simulink model "WorkingDynamics"  (R2018b)
settings: Solver=FixedStepAuto  StartTime=0.0  StopTime=inf  FixedStep=.001  RelTol=5e-3
model workspace (MAT data in the model file):
  A_mu = 10
  B_reff = 8.386
  Cz = 7766.25
  DCT_Param : struct (value not decoded)
  D_reff = 0.25826
  Downshift_Speeds = [9.5625 12.9375 16.3125 19.6875 23.0625 26.4375 29.8125 33.1875 36.5625 39.9375 43.3125 46.6875 ... (28 elements, 4x7)]
  Pedal_Positions = [0.1 0.4 0.5 0.9]
  SUS : struct (value not decoded)
  Upshift_Speeds = [12.9375 16.3125 19.6875 33 26.4375 29.8125 33.1875 52.5 39.9375 43.3125 46.6875 77.25 ... (28 elements, 4x7)]
  VEH : struct (value not decoded)
  V_o = 16.7
  V_xlow = 1
  WH : struct (value not decoded)
  a = 1.4
  alpha_max = 1.5
  alpha_min = -1.5
  b = 1.8
  c_zo = 209651
  epsilon = 0.1
  h = 0.134
  path : struct (value not decoded)
  pio = 220000
  q_Fcx = 0
  q_Fz2 = 15.4
  q_Fzy = 0
  q_reo = 0.9974
  q_sx1 = -0.007764
  q_sx10 = 0.2824
  q_sx11 = 5.349
  q_sx12 = 0
  q_sx13 = 0
  q_sx14 = 0
  q_sx2 = 1.1915
  q_sx3 = 0.013948
  q_sx4 = 4.912
  q_sx5 = 1.02
  q_sx6 = 22.83
  q_sx7 = 0.7104
  q_sx8 = -0.023393
  q_sx9 = 0.6581
  q_sy1 = 0.00702
  q_sy2 = 0
  q_sy3 = 0.001515
  q_sy4 = 8.514e-05
  q_sy5 = 0
  q_sy6 = 0
  q_sy7 = 0.9008
  q_sy8 = -0.4089
  q_v1 = 0.0007742
  q_v2 = 0.04667
  r_Bx1 = 12.531
  r_Bx2 = 9.532
  r_Bx3 = 0
  r_By1 = 10.615
  r_By2 = 7.705
  r_By3 = 3.433e-06
  r_By4 = 0
  r_Cx1 = 1.019
  r_Cy1 = 1.0585
  r_Ex1 = -0.4487
  r_Ex2 = -0.4726
  r_Ey1 = 0.3132
  r_Ey2 = 7.63e-06
  r_Hx1 = 0.0002374
  r_Hy1 = 0.011646
  r_Hy2 = 7.63e-06
  r_Vy1 = 0.05654
  r_Vy2 = 7.63e-06
  r_Vy3 = 0
  r_Vy4 = 99.9
  r_Vy5 = 2
  r_Vy6 = 15.814
  r_o = 0.3135
  vehWidth = 2
  w = 1
libraries: autolibutils x8, autolibshared x6, robotlib x5, simulink x4, autolibsharedcoupling x3, vehdynlibtirecommon x2, sim3dlib x1, vehdynlibsteering x1, autolibshareddiff x1, autolibsharedtransfixedgear x1, sharedtransform x1, autolibsharedmappedengines x1
(part 6 of 6)

== system WorkingDynamics/Passenger Vehicle/Subsystem7/Longitudinal Wheels 4DOF/Veh2Tire ==
  Axle : Inport
  Brake : Inport  Port=2
  r : Inport  Port=3
  VehVel : Inport  Port=4
  WheelSteer : Inport  Port=5
  Reshape3 : Reshape
  Reshape4 : Reshape
  Unary Minus : UnaryMinus
  Wheel to Body Transform : Subsystem
  T : Outport
  P : Outport  Port=2
  xdotAxle : Outport  Port=3
  ydotAxle : Outport  Port=4
  psidot : Outport  Port=5
  zdotAxle : Outport  Port=6
  wires:
  Brake/1 -> Reshape3/1
  Axle/1 -> Reshape4/1
  Wheel to Body Transform/1(xdotWheel) -> xdotAxle/1  "Vx"
  Wheel to Body Transform/2(ydotWheel) -> ydotAxle/1  "Vy"
  r/1 -> Unary Minus/1
  Reshape4/1 -> T/1
  VehVel/1 -> Wheel to Body Transform/1(VelVeh)
  WheelSteer/1 -> Wheel to Body Transform/2(WheelAngles)
  Wheel to Body Transform/3(zdotWheel) -> zdotAxle/1  "Vz"
  Unary Minus/1 -> psidot/1
  Reshape3/1 -> P/1

== system WorkingDynamics/Passenger Vehicle/Subsystem7/Longitudinal Wheels 4DOF/Velocity and Vertical Load ==
  note: 1) Add Subsystem or Model blocks as valid variant choices.
      | 2) You cannot connect blocks at this level. At simulation, connectivity is automatically
      | determined, based on the active variant and port name matching.
  VehFdbk : Inport
  Bicycle : Subsystem  VariantControl=0
  Dual : Subsystem  VariantControl=1
  VehV : Outport
  Fz : Outport  Port=2  PortDimensions=4

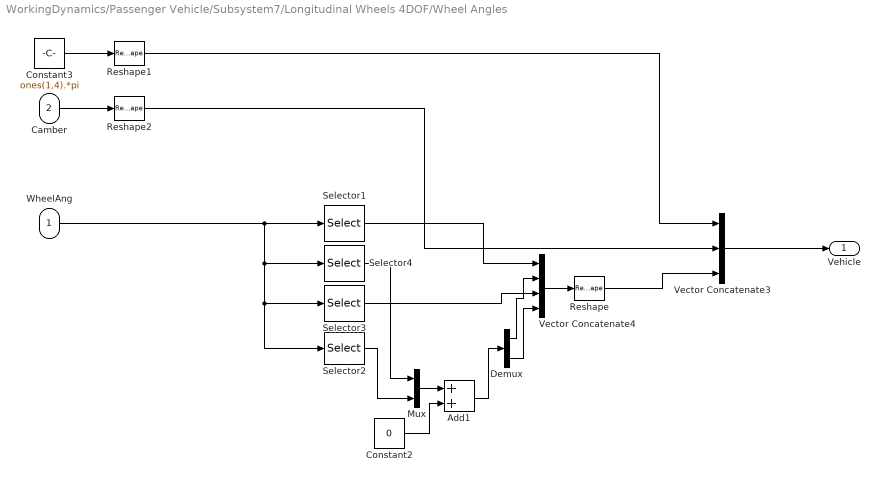
== system WorkingDynamics/Passenger Vehicle/Subsystem7/Longitudinal Wheels 4DOF/Wheel Angles ==
  WheelAng : Inport
  Camber : Inport  Port=2
  Add1 : Sum
  Constant2 : Constant  Value=0
  Constant3 : Constant  Value=ones(1,4).*pi
  Demux : Demux  Outputs=2
  Mux : Mux  Inputs=2
  Reshape : Reshape  OutputDimensionality=Row vector (2-D)
  Reshape1 : Reshape  OutputDimensionality=Row vector (2-D)
  Reshape2 : Reshape  OutputDimensionality=Row vector (2-D)
  Selector1 : Selector  InputPortWidth=4  IndexOptions=Index vector (dialog)  Indices=1  OutputSizes=4
  Selector2 : Selector  InputPortWidth=4  IndexOptions=Index vector (dialog)  Indices=4  OutputSizes=4
  Selector3 : Selector  InputPortWidth=4  IndexOptions=Index vector (dialog)  Indices=3  OutputSizes=4
  Selector4 : Selector  InputPortWidth=4  IndexOptions=Index vector (dialog)  Indices=2  OutputSizes=4
  Vector Concatenate3 : Concatenate  NumInputs=3  Mode=Multidimensional array
  Vector Concatenate4 : Concatenate  NumInputs=4
  Vehicle : Outport
  wires:
  Selector4/1 -> Mux/1
  Constant2/1 -> Add1/2
  Add1/1 -> Demux/1
  Selector3/1 -> Vector Concatenate4/3
  Selector1/1 -> Vector Concatenate4/1
  Mux/1 -> Add1/1
  Selector2/1 -> Mux/2
  Demux/1 -> Vector Concatenate4/2
  Demux/2 -> Vector Concatenate4/4
  Vector Concatenate4/1 -> Reshape/1
  Constant3/1 -> Reshape1/1
  Vector Concatenate3/1 -> Vehicle/1
  Reshape/1 -> Vector Concatenate3/3
  Reshape1/1 -> Vector Concatenate3/1
  Reshape2/1 -> Vector Concatenate3/2
  Camber/1 -> Reshape2/1
  WheelAng/1 -> Selector2/1, Selector3/1, Selector4/1, Selector1/1

== system WorkingDynamics/Vehicle Control/Brake Controller/Brake Pressure Control/Bang Bang ABS ==
  Pref : Inport
  xdot : Inport  Port=2
  <Kappa> : Inport  Port=3
  Abs : Abs
  Add : Sum  Inputs=-+
  Bang-bang controller : Subsystem  mask(Sign){}
      mask help: y = sign(x)
      mask Help: Sign Function:\n\t\t\ty = 1 if x > 0\n\t\t\ty = 0 if x = 0\n\t\t\ty = -1 if x < 0
      mask Display: plot(-50,-50,50,50,[-50,50],[0,0],[0,0],[-50,50],[-40,0],[-30,-30],[0,40],[30,30])
  Compare To Constant : simulink/Logic and Bit Operations/Compare To Constant  relop=>=  const=.2  OutDataTypeStr=boolean
  Compare To Constant1 : simulink/Logic and Bit Operations/Compare To Constant  relop=>=  const=.75  OutDataTypeStr=boolean
  Compare To Constant2 : simulink/Logic and Bit Operations/Compare To Constant  relop=>=  const=.5  OutDataTypeStr=boolean
  Constant : Constant  Value=.25
  Debounce : autolibutils/Debounce  DbcOn_Cnts=.1*.001  DbcOff_Cnts=.1*.001  aMode=aMode
      settings: SourceProductName=Powertrain Blockset  SourceProductBaseCode=PW
  Gain : Gain  Gain=200
  Logical Operator : Logic  Inputs=3  AllPortsSameDT=off  OutDataTypeStr=boolean
  Rate Transition : RateTransition  Deterministic=off  OutPortSampleTime=.001
  Rate Transition1 : RateTransition  Deterministic=off
  Switch : Switch  Criteria=u2 > Threshold  ZeroCross=off
  PCmd : Outport
  wires:
  Bang-bang controller/1(out_1) -> Gain/1
  Add/1 -> Bang-bang controller/1(in_1)
  Rate Transition1/1 -> PCmd/1
  <Kappa>/1 -> Rate Transition/1
  Pref/1 -> Switch/3, Compare To Constant1/1  "Pref"
  Constant/1 -> Add/2  "slip ref"
  Switch/1 -> Rate Transition1/1
  Rate Transition/1 -> Add/1, Compare To Constant/1
  Logical Operator/1 -> Debounce/1
  Compare To Constant/1 -> Logical Operator/2
  Compare To Constant1/1 -> Logical Operator/3
  Debounce/1 -> Switch/2
  xdot/1 -> Abs/1
  Abs/1 -> Compare To Constant2/1
  Compare To Constant2/1 -> Logical Operator/1
  Gain/1 -> Switch/1

== system WorkingDynamics/Vehicle Control/Brake Controller/Brake Pressure Control/Open Loop ==
  Pref : Inport
  PCmd : Outport
  wires:
  Pref/1 -> PCmd/1  "Reference Slip"

== system WorkingDynamics/Vehicle Control/Transmission Controller/TCM/Neutral Select ==
  AccCmd : Inport
  EngSpd : Inport  Port=2
  Constant : Constant  Value=1200
  Constant1 : Constant  Value=1e-6
  Logical Operator : Logic  AllPortsSameDT=off  OutDataTypeStr=boolean
  Relational Operator : RelationalOperator  Operator=<=  OutDataTypeStr=boolean  RndMeth=Simplest
  Relational Operator1 : RelationalOperator  Operator=<=  OutDataTypeStr=boolean  RndMeth=Simplest
  Saturation1 : Saturate  UpperLimit=10e3  LowerLimit=0
  rad/s to RPM : Gain  Gain=30/pi
  Neutral Select : Outport
  wires:
  Saturation1/1 -> Relational Operator/1
  Relational Operator1/1 -> Logical Operator/1
  AccCmd/1 -> Relational Operator1/1
  Constant1/1 -> Relational Operator1/2
  Logical Operator/1 -> Neutral Select/1
  Constant/1 -> Relational Operator/2
  Relational Operator/1 -> Logical Operator/2
  rad/s to RPM/1 -> Saturation1/1
  EngSpd/1 -> rad/s to RPM/1

== system WorkingDynamics/Vehicle Control/Transmission Controller/TCM/TCM Shift Controller/calc ==
  note: Determine if next gear will be
      | higher or lower than current gear
  gear : Inport
  pedal : Inport  Port=2
  speed : Inport  Port=3
  f : TriggerPort  TriggerType=function-call  VariantControl=Variant  StatesWhenEnabling=reset
      settings: CopyFcn=Stateflow.SLINSF.SimulinkMan.removeBlockPreDeleteFcn  PreDeleteFcn=Stateflow.SLINSF.SimulinkMan.unsafePredeleteFcn
  Add1 : Sum  Inputs=+-
  Add3 : Sum  Inputs=+-
  Add4 : Sum  Inputs=+-
  Calculate Upshift Threshold : Lookup_n-D  BreakpointsForDimension1=Pedal_Positions  BreakpointsForDimension2=1:7  Table=Upshift_Speeds  ExtrapMethod=Clip  UseLastTableValue=on  InternalRulePriority=Speed  RndMeth=Simplest  InputSameDT=on
  Calculate Downshift Threshold : Lookup_n-D  BreakpointsForDimension1=Pedal_Positions  BreakpointsForDimension2=2:8  Table=Downshift_Speeds  ExtrapMethod=Clip  UseLastTableValue=on  InternalRulePriority=Speed  RndMeth=Simplest  InputSameDT=on
  SpdThr : Outport
  wires:
  pedal/1 -> Calculate Downshift Threshold/1, Calculate Upshift Threshold/1
  gear/1 -> Calculate Downshift Threshold/2, Calculate Upshift Threshold/2
  Calculate Downshift Threshold/1 -> Add3/2
  Calculate Upshift Threshold/1 -> Add1/1
  speed/1 -> Add1/2, Add3/1
  Add1/1 -> Add4/1
  Add3/1 -> Add4/2
  Add4/1 -> SpdThr/1

== system WorkingDynamics/Vehicle Control/Transmission Controller/TCM/TCM Shift Controller/calc_down ==
  gear : Inport
  pedal : Inport  Port=2
  f : TriggerPort  TriggerType=function-call  VariantControl=Variant  StatesWhenEnabling=reset
      settings: CopyFcn=Stateflow.SLINSF.SimulinkMan.removeBlockPreDeleteFcn  PreDeleteFcn=Stateflow.SLINSF.SimulinkMan.unsafePredeleteFcn
  Calculate Downshift Threshold : Lookup_n-D  BreakpointsForDimension1=Pedal_Positions  BreakpointsForDimension2=2:8  Table=Downshift_Speeds  ExtrapMethod=Clip  UseLastTableValue=on  InternalRulePriority=Speed  RndMeth=Simplest  InputSameDT=on
  down_th : Outport
  wires:
  Calculate Downshift Threshold/1 -> down_th/1
  gear/1 -> Calculate Downshift Threshold/2
  pedal/1 -> Calculate Downshift Threshold/1

== system WorkingDynamics/Vehicle Control/Transmission Controller/TCM/TCM Shift Controller/calc_up ==
  gear : Inport
  pedal : Inport  Port=2
  f : TriggerPort  TriggerType=function-call  VariantControl=Variant  StatesWhenEnabling=reset
      settings: CopyFcn=Stateflow.SLINSF.SimulinkMan.removeBlockPreDeleteFcn  PreDeleteFcn=Stateflow.SLINSF.SimulinkMan.unsafePredeleteFcn
  Calculate Upshift Threshold : Lookup_n-D  BreakpointsForDimension1=Pedal_Positions  BreakpointsForDimension2=1:7  Table=Upshift_Speeds  ExtrapMethod=Clip  UseLastTableValue=on  InternalRulePriority=Speed  RndMeth=Simplest  InputSameDT=on
  up_th : Outport
  wires:
  Calculate Upshift Threshold/1 -> up_th/1
  pedal/1 -> Calculate Upshift Threshold/1
  gear/1 -> Calculate Upshift Threshold/2

== system WorkingDynamics/Passenger Vehicle/Subsystem7/Longitudinal Wheels 4DOF/Axle Forces/Bicycle ==
  F : Inport
  R : Inport  Port=2
  Sum of Elements : Sum  Inputs=+
  Sum of Elements1 : Sum  Inputs=+
  FrntAxlF : Outport  Unit=N
  RearAxlF : Outport  Port=2  Unit=N
  wires:
  Sum of Elements/1 -> FrntAxlF/1
  Sum of Elements1/1 -> RearAxlF/1
  R/1 -> Sum of Elements1/1
  F/1 -> Sum of Elements/1

== system WorkingDynamics/Passenger Vehicle/Subsystem7/Longitudinal Wheels 4DOF/Axle Forces/Dual ==
  F : Inport
  R : Inport  Port=2
  FrntAxlF : Outport  Unit=N
  RearAxlF : Outport  Port=2  Unit=N
  wires:
  R/1 -> RearAxlF/1
  F/1 -> FrntAxlF/1

== system WorkingDynamics/Passenger Vehicle/Subsystem7/Longitudinal Wheels 4DOF/Tires/Fx ==
  In1 : Inport
  In2 : Inport  Port=2
  In3 : Inport  Port=3
  In4 : Inport  Port=4
  Bus Selector{,1..3} (4 alike) : BusSelector  OutputSignals=Fx
  Vector Concatenate : Concatenate  NumInputs=4
  Out1 : Outport
  wires:
  Bus Selector3/1 -> Vector Concatenate/4  "<Fx>"
  Bus Selector2/1 -> Vector Concatenate/3  "<Fx>"
  Bus Selector1/1 -> Vector Concatenate/2  "<Fx>"
  In4/1 -> Bus Selector3/1
  In3/1 -> Bus Selector2/1
  In2/1 -> Bus Selector1/1
  Bus Selector/1 -> Vector Concatenate/1  "<Fx>"
  In1/1 -> Bus Selector/1
  Vector Concatenate/1 -> Out1/1

== system WorkingDynamics/Passenger Vehicle/Subsystem7/Longitudinal Wheels 4DOF/Tires/Fz1 ==
  In1 : Inport
  In2 : Inport  Port=2
  In3 : Inport  Port=3
  In4 : Inport  Port=4
  Bus Selector{,1..3} (4 alike) : BusSelector  OutputSignals=Fz
  Vector Concatenate : Concatenate  NumInputs=4
  Out1 : Outport
  wires:
  Vector Concatenate/1 -> Out1/1
  In1/1 -> Bus Selector/1
  Bus Selector/1 -> Vector Concatenate/1  "<Fz>"
  In2/1 -> Bus Selector1/1
  In3/1 -> Bus Selector2/1
  In4/1 -> Bus Selector3/1
  Bus Selector1/1 -> Vector Concatenate/2  "<Fz>"
  Bus Selector2/1 -> Vector Concatenate/3  "<Fz>"
  Bus Selector3/1 -> Vector Concatenate/4  "<Fz>"

== system WorkingDynamics/Passenger Vehicle/Subsystem7/Longitudinal Wheels 4DOF/Tires/My ==
  In1 : Inport
  In2 : Inport  Port=2
  In3 : Inport  Port=3
  In4 : Inport  Port=4
  Bus Selector{,1..3} (4 alike) : BusSelector  OutputSignals=My
  Vector Concatenate : Concatenate  NumInputs=4
  Out1 : Outport  PortDimensions=4
  wires:
  Bus Selector3/1 -> Vector Concatenate/4  "<My>"
  Bus Selector2/1 -> Vector Concatenate/3  "<My>"
  Bus Selector1/1 -> Vector Concatenate/2  "<My>"
  In4/1 -> Bus Selector3/1
  In3/1 -> Bus Selector2/1
  In2/1 -> Bus Selector1/1
  Bus Selector/1 -> Vector Concatenate/1  "<My>"
  In1/1 -> Bus Selector/1
  Vector Concatenate/1 -> Out1/1

== system WorkingDynamics/Passenger Vehicle/Subsystem7/Longitudinal Wheels 4DOF/Tires/Re ==
  In1 : Inport
  In2 : Inport  Port=2
  In3 : Inport  Port=3
  In4 : Inport  Port=4
  Bus Selector{,1..3} (4 alike) : BusSelector  OutputSignals=Re
  Vector Concatenate : Concatenate  NumInputs=4
  Out1 : Outport  PortDimensions=4
  wires:
  Vector Concatenate/1 -> Out1/1
  In1/1 -> Bus Selector/1
  Bus Selector/1 -> Vector Concatenate/1  "<Re>"
  In2/1 -> Bus Selector1/1
  In3/1 -> Bus Selector2/1
  In4/1 -> Bus Selector3/1
  Bus Selector1/1 -> Vector Concatenate/2  "<Re>"
  Bus Selector2/1 -> Vector Concatenate/3  "<Re>"
  Bus Selector3/1 -> Vector Concatenate/4  "<Re>"

== system WorkingDynamics/Passenger Vehicle/Subsystem7/Longitudinal Wheels 4DOF/Tires/alpha ==
  In1 : Inport
  In2 : Inport  Port=2
  In3 : Inport  Port=3
  In4 : Inport  Port=4
  Vector Concatenate : Concatenate  NumInputs=4
  Out1 : Outport  PortDimensions=4
  wires:
  Vector Concatenate/1 -> Out1/1
  In1/1 -> Vector Concatenate/1
  In2/1 -> Vector Concatenate/2
  In3/1 -> Vector Concatenate/3
  In4/1 -> Vector Concatenate/4

== system WorkingDynamics/Passenger Vehicle/Subsystem7/Longitudinal Wheels 4DOF/Tires/kappa ==
  In1 : Inport
  In2 : Inport  Port=2
  In3 : Inport  Port=3
  In4 : Inport  Port=4
  Bus Selector{,1..3} (4 alike) : BusSelector  OutputSignals=Kappa
  Vector Concatenate : Concatenate  NumInputs=4
  Out1 : Outport  PortDimensions=4
  wires:
  Bus Selector3/1 -> Vector Concatenate/4  "<Kappa>"
  Bus Selector2/1 -> Vector Concatenate/3  "<Kappa>"
  Bus Selector1/1 -> Vector Concatenate/2  "<Kappa>"
  In4/1 -> Bus Selector3/1
  In3/1 -> Bus Selector2/1
  In2/1 -> Bus Selector1/1
  Bus Selector/1 -> Vector Concatenate/1  "<Kappa>"
  In1/1 -> Bus Selector/1
  Vector Concatenate/1 -> Out1/1

== system WorkingDynamics/Passenger Vehicle/Subsystem7/Longitudinal Wheels 4DOF/Tires/omega ==
  In1 : Inport
  In2 : Inport  Port=2
  In3 : Inport  Port=3
  In4 : Inport  Port=4
  Bus Selector{1..4} (4 alike) : BusSelector  OutputSignals=Omega
  Vector Concatenate : Concatenate  NumInputs=4
  Out1 : Outport
  wires:
  In1/1 -> Bus Selector4/1
  Bus Selector4/1 -> Vector Concatenate/1  "<Omega>"
  In2/1 -> Bus Selector2/1
  In3/1 -> Bus Selector1/1
  In4/1 -> Bus Selector3/1
  Bus Selector2/1 -> Vector Concatenate/2  "<Omega>"
  Bus Selector1/1 -> Vector Concatenate/3  "<Omega>"
  Bus Selector3/1 -> Vector Concatenate/4  "<Omega>"
  Vector Concatenate/1 -> Out1/1

== system WorkingDynamics/Passenger Vehicle/Subsystem7/Longitudinal Wheels 4DOF/Tires/z ==
  In1 : Inport
  In2 : Inport  Port=2
  In3 : Inport  Port=3
  In4 : Inport  Port=4
  Bus Selector{,1..3} (4 alike) : BusSelector  OutputSignals=z
  Vector Concatenate : Concatenate  NumInputs=4
  Out1 : Outport  PortDimensions=4
  wires:
  Bus Selector3/1 -> Vector Concatenate/4  "<z>"
  Bus Selector2/1 -> Vector Concatenate/3  "<z>"
  Bus Selector1/1 -> Vector Concatenate/2  "<z>"
  In4/1 -> Bus Selector3/1
  In3/1 -> Bus Selector2/1
  In2/1 -> Bus Selector1/1
  Bus Selector/1 -> Vector Concatenate/1  "<z>"
  In1/1 -> Bus Selector/1
  Vector Concatenate/1 -> Out1/1

== system WorkingDynamics/Passenger Vehicle/Subsystem7/Longitudinal Wheels 4DOF/Tires/zdot ==
  In1 : Inport
  In2 : Inport  Port=2
  In3 : Inport  Port=3
  In4 : Inport  Port=4
  Bus Selector{,1..3} (4 alike) : BusSelector  OutputSignals=zdot
  Vector Concatenate : Concatenate  NumInputs=4
  Out1 : Outport  PortDimensions=4
  wires:
  Vector Concatenate/1 -> Out1/1
  In1/1 -> Bus Selector/1
  Bus Selector/1 -> Vector Concatenate/1  "<zdot>"
  In2/1 -> Bus Selector1/1
  In3/1 -> Bus Selector2/1
  In4/1 -> Bus Selector3/1
  Bus Selector1/1 -> Vector Concatenate/2  "<zdot>"
  Bus Selector2/1 -> Vector Concatenate/3  "<zdot>"
  Bus Selector3/1 -> Vector Concatenate/4  "<zdot>"

== system WorkingDynamics/Passenger Vehicle/Subsystem7/Longitudinal Wheels 4DOF/Veh2Tire/Wheel to Body Transform ==
  VelVeh : Inport  Partition=on  PartitionDimension=2  PartitionWidth=1  PartitionOffset=0
  WheelAngles : Inport  Port=2  Partition=on  PartitionDimension=2  PartitionWidth=1  PartitionOffset=0
  Demux1 : Demux  Outputs=3
  Divide1 : Product  Inputs=**  Multiplication=Matrix(*)
  For Each : ForEach  DisableCoverage=on  IndexMode=One-based
  Rotation Angles to Direction Cosine Matrix : sharedtransform/Rotation Angles to Direction Cosine Matrix  rotationOrder=ZYX  aMode=2
      settings: SourceProductBaseCode=AE
  Selector : Selector  InputPortWidth=3  IndexOptions=Index vector (dialog)  Indices=[3 2 1]  OutputSizes=1
  xdotWheel : Outport  ConcatenationDimension=1
  ydotWheel : Outport  Port=2  ConcatenationDimension=1
  zdotWheel : Outport  Port=3  ConcatenationDimension=1
  wires:
  Divide1/1 -> Demux1/1
  Demux1/1 -> xdotWheel/1
  Demux1/2 -> ydotWheel/1
  Demux1/3 -> zdotWheel/1
  Rotation Angles to Direction Cosine Matrix/1 -> Divide1/1
  VelVeh/1 -> Divide1/2
  WheelAngles/1 -> Selector/1
  Selector/1 -> Rotation Angles to Direction Cosine Matrix/1

== system WorkingDynamics/Passenger Vehicle/Subsystem7/Longitudinal Wheels 4DOF/Velocity and Vertical Load/Bicycle ==
  VehFdbk : Inport
  Bicycle Fz : Subsystem
  Bicycle V : Subsystem
  VehV : Outport
  Fz : Outport  Port=2
  wires:
  Bicycle V/1(Out1) -> VehV/1
  Bicycle Fz/1(Out1) -> Fz/1
  VehFdbk/1 -> Bicycle Fz/1(In1), Bicycle V/1(In1)

== system WorkingDynamics/Passenger Vehicle/Subsystem7/Longitudinal Wheels 4DOF/Velocity and Vertical Load/Dual ==
  VehFdbk : Inport
  Dual Fz : Subsystem
  Dual V : Subsystem
  VehV : Outport
  Fz : Outport  Port=2
  wires:
  Dual V/1(Out1) -> VehV/1
  VehFdbk/1 -> Dual Fz/1(In1), Dual V/1(In1)
  Dual Fz/1(Out1) -> Fz/1

== system WorkingDynamics/Vehicle Control/Brake Controller/Brake Pressure Control/Bang Bang ABS/Bang-bang controller ==
  in_1 : Inport
  Constant : Constant  Value=0
  Data Type Conversion1 : DataTypeConversion  OutDataTypeStr=double  SaturateOnIntegerOverflow=on  RndMeth=Zero
  Data Type Conversion2 : DataTypeConversion  OutDataTypeStr=double  SaturateOnIntegerOverflow=on  RndMeth=Zero
  Relational Operator : RelationalOperator  Operator=>  OutDataTypeStr=boolean  RndMeth=Nearest  InputSameDT=on
  Relational Operator1 : RelationalOperator  Operator=<  OutDataTypeStr=boolean  RndMeth=Nearest  InputSameDT=on
  Sum : Sum  Inputs=+-  SaturateOnIntegerOverflow=on  InputSameDT=on  OutDataTypeStr=Inherit: Same as first input
  out_1 : Outport  InitialOutput=0
  wires:
  Data Type Conversion2/1 -> Sum/2
  Data Type Conversion1/1 -> Sum/1
  Sum/1 -> out_1/1
  Relational Operator/1 -> Data Type Conversion1/1
  Relational Operator1/1 -> Data Type Conversion2/1
  Constant/1 -> Relational Operator/2, Relational Operator1/2
  in_1/1 -> Relational Operator1/1, Relational Operator/1

== system WorkingDynamics/Passenger Vehicle/Subsystem7/Longitudinal Wheels 4DOF/Velocity and Vertical Load/Bicycle/Bicycle Fz ==
  In1 : Inport
  Bus Selector6 : BusSelector  OutputSignals=BdyFrm.Forces.Tires.FrntTire.Fz,BdyFrm.Forces.Tires.RearTire.Fz
  Cont LPF : autolibutils/Cont LPF  wc=20*2*pi  aMode=2
      settings: SourceProductName=Powertrain Blockset  SourceProductBaseCode=PW
  Mux5 : Mux
  Saturation : Saturate  UpperLimit=20e3  LowerLimit=1000  ZeroCross=off
  Out1 : Outport
  wires:
  Cont LPF/1 -> Out1/1
  Saturation/1 -> Cont LPF/1
  Bus Selector6/2 -> Mux5/4, Mux5/3  "<Fz>"
  In1/1 -> Bus Selector6/1
  Bus Selector6/1 -> Mux5/2, Mux5/1  "<Fz>"
  Mux5/1 -> Saturation/1

== system WorkingDynamics/Passenger Vehicle/Subsystem7/Longitudinal Wheels 4DOF/Velocity and Vertical Load/Bicycle/Bicycle V ==
  In1 : Inport
  Bus Selector : BusSelector  OutputSignals=BdyFrm.FrntAxl.Vel.xdot,BdyFrm.FrntAxl.Vel.ydot,BdyFrm.FrntAxl.Vel.zdot  OutputAsBus=on
  Bus Selector3 : BusSelector  OutputSignals=BdyFrm.RearAxl.Vel.xdot,BdyFrm.RearAxl.Vel.ydot,BdyFrm.RearAxl.Vel.zdot  OutputAsBus=on
  Bus to Vector1 : BusToVector
  Bus to Vector3 : BusToVector
  Vector Concatenate1 : Concatenate  NumInputs=4  Mode=Multidimensional array  ConcatenateDimension=2
  Out1 : Outport
  wires:
  Bus Selector3/1 -> Bus to Vector3/1
  Bus to Vector1/1 -> Vector Concatenate1/2, Vector Concatenate1/1
  In1/1 -> Bus Selector3/1, Bus Selector/1
  Bus Selector/1 -> Bus to Vector1/1
  Bus to Vector3/1 -> Vector Concatenate1/4, Vector Concatenate1/3
  Vector Concatenate1/1 -> Out1/1

== system WorkingDynamics/Passenger Vehicle/Subsystem7/Longitudinal Wheels 4DOF/Velocity and Vertical Load/Dual/Dual Fz ==
  In1 : Inport
  Bus Selector6 : BusSelector  OutputSignals=BdyFrm.Forces.Tires.FrntTires.Lft.Fz,BdyFrm.Forces.Tires.FrntTires.Rght.Fz,BdyFrm.Forces.Tires.RearTires.Lft.Fz,BdyFrm.Forces.Tires.RearTires.Rght.Fz
  Cont LPF : autolibutils/Cont LPF  wc=20*2*pi  aMode=2
      settings: SourceProductName=Powertrain Blockset  SourceProductBaseCode=PW
  Saturation : Saturate  UpperLimit=20e3  LowerLimit=1000  ZeroCross=off
  Vector Concatenate : Concatenate  NumInputs=4
  Out1 : Outport
  wires:
  In1/1 -> Bus Selector6/1
  Saturation/1 -> Cont LPF/1
  Cont LPF/1 -> Out1/1
  Vector Concatenate/1 -> Saturation/1
  Bus Selector6/2 -> Vector Concatenate/2  "<Fz>"
  Bus Selector6/1 -> Vector Concatenate/1  "<Fz>"
  Bus Selector6/3 -> Vector Concatenate/3  "<Fz>"
  Bus Selector6/4 -> Vector Concatenate/4  "<Fz>"

== system WorkingDynamics/Passenger Vehicle/Subsystem7/Longitudinal Wheels 4DOF/Velocity and Vertical Load/Dual/Dual V ==
  In1 : Inport
  Bus Selector1 : BusSelector  OutputSignals=BdyFrm.FrntAxl.Lft.Vel.xdot,BdyFrm.FrntAxl.Lft.Vel.ydot,BdyFrm.FrntAxl.Lft.Vel.zdot  OutputAsBus=on
  Bus Selector2 : BusSelector  OutputSignals=BdyFrm.FrntAxl.Rght.Vel.xdot,BdyFrm.FrntAxl.Rght.Vel.ydot,BdyFrm.FrntAxl.Rght.Vel.zdot  OutputAsBus=on
  Bus Selector4 : BusSelector  OutputSignals=BdyFrm.RearAxl.Lft.Vel.xdot,BdyFrm.RearAxl.Lft.Vel.ydot,BdyFrm.RearAxl.Lft.Vel.zdot  OutputAsBus=on
  Bus Selector5 : BusSelector  OutputSignals=BdyFrm.RearAxl.Rght.Vel.xdot,BdyFrm.RearAxl.Rght.Vel.ydot,BdyFrm.RearAxl.Rght.Vel.zdot  OutputAsBus=on
  Bus to Vector{5..8} (4 alike) : BusToVector
  Vector Concatenate2 : Concatenate  NumInputs=4  Mode=Multidimensional array  ConcatenateDimension=2
  Out1 : Outport
  wires:
  Bus to Vector6/1 -> Vector Concatenate2/2
  Bus Selector2/1 -> Bus to Vector6/1
  Bus to Vector8/1 -> Vector Concatenate2/4
  Bus Selector4/1 -> Bus to Vector7/1
  Bus to Vector5/1 -> Vector Concatenate2/1
  Bus Selector1/1 -> Bus to Vector5/1
  In1/1 -> Bus Selector1/1, Bus Selector2/1, Bus Selector4/1, Bus Selector5/1
  Bus Selector5/1 -> Bus to Vector8/1
  Bus to Vector7/1 -> Vector Concatenate2/3
  Vector Concatenate2/1 -> Out1/1

== stateflow chart WorkingDynamics/Vehicle Control/Transmission Controller/TCM/TCM Shift Controller ==
  settings: sampleTime=0.01
  state GearState [parallel]
    settings: executionOrder=1
    state Neutral
      en:
      GearState = 0;
    state G1
      en:
      GearState = 1;
    state G2
      en:
      GearState = 2;
      du:
      [SpdThr] = calc(2,pedal,speed);
    state G3
      en:
      GearState = 3;
      du:
      [SpdThr] = calc(3,pedal,speed);
    state G8
      en:
      GearState = 8;
    state G7
      en:
      GearState = 7;
    state G6
      en:
      GearState = 6;
    state G5
      en:GearState=5;
      du:[SpdThr]=calc(5,pedal,speed);
    state G4
      en:
      GearState = 4;
      du:
      [SpdThr] = calc(4,pedal,speed);
    (default) -> G1
    Neutral -> G1 : [~Neutral]
    G1 -> G2 [order 1] : Up
    G2 -> G3 [order 1] : Up
    G1 -> Neutral [order 2] : [Neutral]
    G2 -> G1 [order 2] : Down
    G3 -> G2 [order 2] : Down
    G3 -> G4 [order 1] : Up
    G4 -> G3 [order 2] : Down
    G7 -> G8 [order 1] : Up
    G5 -> G6 [order 1] : Up
    G6 -> G7 [order 1] : Up
    G4 -> G5 [order 1] : Up
    G5 -> G4 [order 2] : Down
    G6 -> G5 [order 2] : Down
    G7 -> G6 [order 2] : Down
    G8 -> G7 : Down
  state SelectionState [parallel]
    du:[up_th]=calc_up(GearState,pedal);
    du:[down_th]=calc_down(GearState,pedal);
    settings: executionOrder=2
    state SteadyState
      en:
      clutchControl = 0;
    state preDownShifting
    state preUpShifting
    state UpShifting
      en:
      GearState = GearState + 0.5;
    state DownShifting
      en:
      GearState = GearState - 0.5;
    (default) -> SteadyState
    SteadyState -> (junction 62) [order 1] : [speed < down_th && ...
        | GearState >1]
    SteadyState -> (junction 128) [order 2] : [speed > up_th &&...
        | GearState <= 5 && ...
        | floor(GearState) == GearState]
    (junction 62) -> preDownShifting
    (junction 128) -> preUpShifting
    (junction 168) -> SteadyState
    (junction 23) -> SteadyState
    (junction 161) -> SteadyState
    preDownShifting -> (junction 168) [order 2] : [speed >= down_th]
    preUpShifting -> (junction 161) [order 2] : [speed <= up_th]
    preUpShifting -> UpShifting [order 1] : after(0.5,sec)
        | [speed>up_th]
    preDownShifting -> DownShifting [order 1] : after(0.5, sec)
        | [speed < down_th - 2]
    DownShifting -> (junction 23) : {GearState.Down;}
    UpShifting -> (junction 23) : {GearState.Up;}
  state up_th = calc_up(gear,pedal) [function]
  state down_th = calc_down(gear,pedal) [function]
  state SpdThr = calc(gear,pedal,speed) [function]
  data: gear function_input; pedal function_input; up_th function_output; gear function_input; pedal function_input; down_th function_output; gear function_input; pedal function_input; SpdThr function_output; speed function_input; GearState output int8; speed input; pedal input; clutchControl local double; SpdThr local double; Neutral input; up_th local double; down_th local double
  events: Up local EITHER_EDGE_EVENT; Down local EITHER_EDGE_EVENT

== matlab function WorkingDynamics/Dead Man's Switch/timeout set to 0 output ==
  data: isNew input; safeValue output; value input; timeout input; timedOut output; stepSize input
function [safeValue,timedOut] = fcn(isNew,value,timeout,stepSize)
%#codegen
persistent sinceLastMsg
timedOut=true;
if isempty(sinceLastMsg)
    sinceLastMsg=(timeout/stepSize)+1;
end

safeValue=0;
% if no new message
% after timeout, we output 0
if( isNew == true )
    sinceLastMsg = 0;
else
    sinceLastMsg = sinceLastMsg+1;
end

% Note: we require step size as an input here, and depend on our
% system being executed at a regular rate, or bad things will happen
if( sinceLastMsg < timeout/stepSize )
    timedOut = false;
end
    
if( timedOut == false )
    safeValue = value;
end
